simulink model "HIL_HallTesting"  (R2024b)
settings: Solver=ode23t  StartTime=0.0  StopTime=Inf  FixedStep=1e-2  RelTol=1e-3
undefined symbols (not defined in the file): DiscIntNeverNeededParam
libraries: fl_lib x6, nesl_utility x4, instrumentseriallib x3, svdutilitieslib x2
settings Model: SimulationMode=accelerator  Creator=luigi  LastModifiedBy=luigi
settings HardwareCC: ProdBitPerLong=64  ProdHWDeviceType=Intel->x86-64 (Linux 64)
settings SFSimCC: SimCustomCompilerFlags="CFLAGS  = -g -Wall -std=c99 -D_POSIX_SOURCE -D_GNU_SOURCE LDFLAGS = -lpthread -lrt"
settings RTWCC: Description=Simulink Desktop Real-Time  SystemTargetFile=sldrt.tlc  GenerateMakefile=off  TemplateMakefile=sldrt.tmf  CustomInclude=/usr/include/linux/  RTWCompilerOptimization=on
settings RTWCC: CustomHeaderCode=|
  | #include "time.h"
  | #include "stdint.h"
settings CodeAppCC: MaxIdLength=95
settings SimulinkDesktopRealTimeCC: TargetLibSuffix=_sldrt.a  TargetPreCompLibLocation=/usr/local/MATLAB/R2024b/toolbox/sldrt/lib/glnxa64  CodeReplacementLibrary=GNU C99 extensions  ParMdlRefBuildCompliant=on

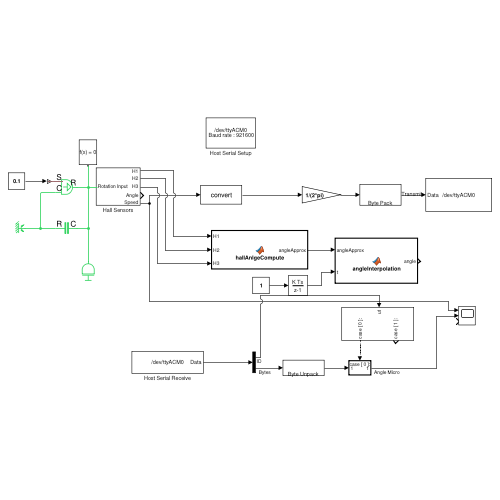
[thumbnail: Simulink's stored preview of the top-level diagram]
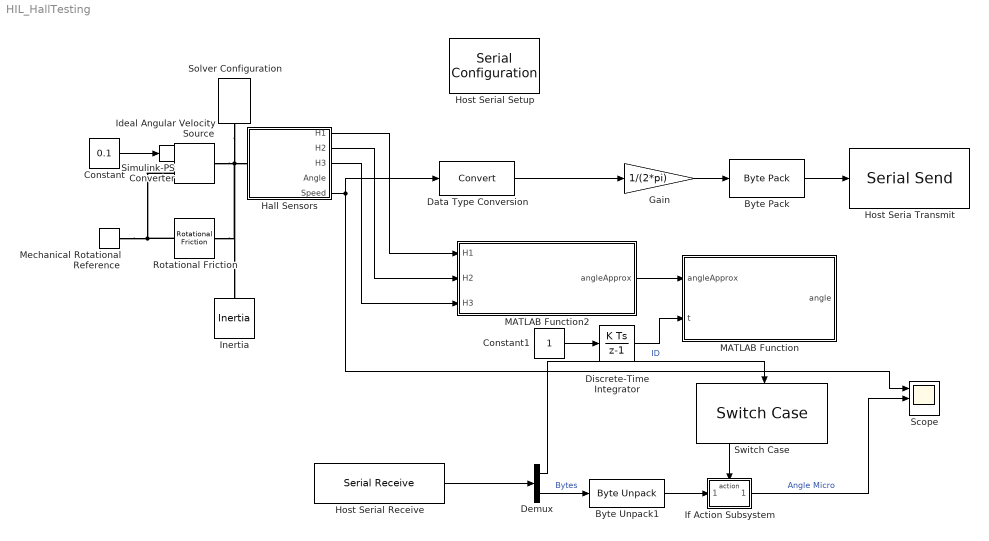
== system HIL_HallTesting ==
  Byte Pack : svdutilitieslib/Byte Pack  maskPackedDataType=uint8  datatypes={'single'}  byteAlign=1  blockPlatform=arduinoert
      settings: LibrarySourceBlock=mcblib/Signal Management/Byte Pack
  Byte Unpack1 : svdutilitieslib/Byte Unpack  dimensions={[1]}  datatypes={'single'}  byteAlign=1  blockPlatform=arduinoert
      settings: LibrarySourceBlock=mcblib/Signal Management/Byte Unpack
  Constant : Constant  Value=0.1
  Constant1 : Constant
  Data Type Conversion : DataTypeConversion  SaturateOnIntegerOverflow=off  RndMeth=Floor
  Demux : Demux  Outputs=[1 4]
  Discrete-Time Integrator : DiscreteIntegrator  SampleTime=-1  ICPrevOutput=DiscIntNeverNeededParam  ICPrevScaledInput=DiscIntNeverNeededParam
  Gain : Gain  Gain=1/(2*pi)
  Hall Sensors : Subsystem
  Host Seria Transmit : instrumentseriallib/Serial Send  PortSel=/dev/ttyACM0  Port=/dev/ttyACM0  ComPort=/dev/ttyACM0  Header=6  Terminator=<none>  CustomTerminator='EOF'  EnableBlockingMode=off  SimulateUsing=Interpreted execution  BlockInModel=on  aMode=5
      settings: LibrarySourceBlock=mcblib/Protection and Diagnostics/Host Serial Transmit
  Host Serial Receive : instrumentseriallib/Serial Receive  PortSel=/dev/ttyACM0  Port=/dev/ttyACM0  ComPort=/dev/ttyACM0  DataType=uint8  SaveDataType=uint8  ToggleHeader=off  Header='S'  ToggleDataSize=on  DataSize=5  ToggleTerminator=on  Terminator=Custom terminator  CustomTerminator='EOF'  InputFormat=Column major  EnableBlockingMode=on  ActionDataUnavailable=Output last received value  ActionWhenDataUnavailable=Output last received value  CustomValue=0  SampleTime=1e-2  SimulateUsing=Interpreted execution  BlockInModel=on  aMode=5
      settings: LibrarySourceBlock=mcblib/Protection and Diagnostics/Host Serial Receive
  Host Serial Setup : instrumentseriallib/Serial Configuration  Priority=-99  PortSel=/dev/ttyACM0  Port=/dev/ttyACM0  ComPort=/dev/ttyACM0  BaudRate=921600  DataBits=8  Parity=none  StopBits=1  ByteOrder=little-endian  FlowControl=none  Timeout=10  SimulateUsing=Interpreted execution  BlockInModel=on  aMode=5
      settings: LibrarySourceBlock=mcblib/Protection and Diagnostics/Host Serial Setup
  Ideal Angular Velocity Source : fl_lib/Mechanical/Mechanical Sources/Ideal Angular Velocity Source
  If Action Subsystem : Subsystem  TreatAsAtomicUnit=on
  Inertia : fl_lib/Mechanical/Rotational Elements/Inertia  inertia=0.1 kg*m^2  num_ports=foundation.enum.numPorts2.one  w_specify=off  w_priority=High  w=0 rad/s  w_nominal_specify=off  w_nominal_value=1  w_nominal_unit=rad/s  t_specify=off  t_priority=None  t=0 N*m  t_nominal_specify=off  t_nominal_value=1  t_nominal_unit=N*m
  MATLAB Function : MATLAB Function  TreatAsAtomicUnit=on  SystemSampleTime=1e-3
  MATLAB Function2 : MATLAB Function  TreatAsAtomicUnit=on
  Mechanical Rotational Reference : fl_lib/Mechanical/Rotational Elements/Mechanical Rotational Reference
  Rotational Friction : fl_lib/Mechanical/Rotational Elements/Rotational Friction  brkwy_trq=0.05 N*m  brkwy_vel=0.1 rad/s  Col_trq=0.01 N*m  visc_coef=0.01 N*m*s/rad  w_specify=off  w_priority=None  w=0 rad/s  w_nominal_specify=off  w_nominal_value=1  w_nominal_unit=rad/s  t_specify=off  t_priority=None  t=0 N*m  t_nominal_specify=off  t_nominal_value=1  t_nominal_unit=N*m
  Scope : Scope  NumInputPorts=3
  Simulink-PS Converter : nesl_utility/Simulink-PS Converter  PhysicalDomain=network_engine_domain  SubClassName=ps_input  LeftPortType=input  RightPortType=output  PseudoPeriodic=off  Frequencies=[]  NoiseDistribution=none  NoiseParameters=[]  Unit=1  AffineConversion=off  FilteringAndDerivatives=provide  SimscapeFilterOrder=1  InputFilterTimeConstant=0.001  UdotUserProvided=0
  Solver Configuration : nesl_utility/Solver Configuration  PhysicalDomain=network_engine_domain  SubClassName=solver  LeftPortType=input  RightPortType=generic  Tones=[]  Harmonics=[]  SimulateNoise=off  Profile=off  UseLocalSampling=off  EnableSwitchedLinearOptims=on  FrequencyDomain=off  UseCCode=off  RelTol=0.001  AbsTol=0.001  MinStep=1e-09  ToWorkspace=off  RevertToSquareIcSolve=off  NumHomotopyIterations=100  PhasorMode=off  PhasorModeNumHarmonics=1  ConsistencySolver=NEWTON_XTOL_AFTER_FTOL  IndexReductionMethod=DerivativeReplacement  DoDC=off  ResidualTolerance=1e-09  ConsistencyTolSource=GLOBAL  ConsistencyAbsTol=0.001  ConsistencyRelTol=0.001  ConsistencyTolFactor=0.001  UseLocalSolver=off  LocalSolverChoice=NE_BACKWARD_EULER_ADVANCER  ResolveIndetEquations=on  FunctionEvalNumThread=1  LocalSolverSampleTime=0.001  DoFixedCost=off  MaxNonlinIter=3  MaxModeIter=2  ComputeImpulses=off  ImpulseIterations=2  LinearAlgebra=auto  LinearAlgebraNumThread=0  EquationFormulation=NE_TIME_EF  DelaysMemoryBudget=1024  AutomaticFiltering=on  FilteringTimeConstant=0.001  PartitionStorageMethod=AS_NEEDED  PartitionMemoryBudget=1024  PartitionMethod=ROBUST  MultibodyUseLocalSolver=off  MultibodyLocalSolverChoice=ODE1  MultibodyLocalSolverSampleTime=0.001
  Switch Case : SwitchCase  CaseConditions={0,1}  ShowDefaultCase=off
  wires:
  Constant/1 -> Simulink-PS Converter/1
  Hall Sensors/1(H1) -> MATLAB Function2/1(H1)
  Hall Sensors/2(H2) -> MATLAB Function2/2(H2)
  Hall Sensors/3(H3) -> MATLAB Function2/3(H3)
  Discrete-Time Integrator/1 -> MATLAB Function/2(t)
  MATLAB Function2/1(angleApprox) -> MATLAB Function/1(angleApprox)
  Host Serial Receive/1 -> Demux/1
  Demux/1 -> Switch Case/1  "ID"
  Switch Case/1 -> If Action Subsystem/Action
  Byte Unpack1/1 -> If Action Subsystem/1(In1)
  Demux/2 -> Byte Unpack1/1  "Bytes"
  If Action Subsystem/1(Out1) -> Scope/2  "Angle Micro"
  Constant1/1 -> Discrete-Time Integrator/1
  Hall Sensors/5(Speed) -> Data Type Conversion/1, Scope/1
  Byte Pack/1 -> Host Seria Transmit/1
  Gain/1 -> Byte Pack/1
  Data Type Conversion/1 -> Gain/1
  connections:
  Mechanical Rotational Reference/LConn1 -- Ideal Angular Velocity Source/RConn2 -- Rotational Friction/LConn1
  Ideal Angular Velocity Source/RConn1 -- Simulink-PS Converter/RConn1
  Solver Configuration/RConn1 -- Ideal Angular Velocity Source/LConn1 -- Rotational Friction/RConn1 -- Inertia/LConn1 -- Hall Sensors/LConn1

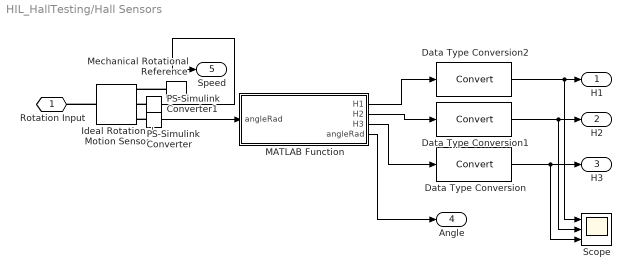
== system HIL_HallTesting/Hall Sensors ==
  Data Type Conversion : DataTypeConversion  SaturateOnIntegerOverflow=off  RndMeth=Floor
  Data Type Conversion1 : DataTypeConversion  SaturateOnIntegerOverflow=off  RndMeth=Floor
  Data Type Conversion2 : DataTypeConversion  SaturateOnIntegerOverflow=off  RndMeth=Floor
  Ideal Rotational Motion Sensor : fl_lib/Mechanical/Mechanical Sensors/Ideal Rotational Motion Sensor  reference=foundation.enum.MeasurementReference.difference  acceleration_port=false  velocity_port=true  position_port=true  wrap_angle=true  offset=0 rad
  MATLAB Function : MATLAB Function  TreatAsAtomicUnit=on
  Mechanical Rotational Reference : fl_lib/Mechanical/Rotational Elements/Mechanical Rotational Reference
  PS-Simulink Converter : nesl_utility/PS-Simulink Converter  PhysicalDomain=network_engine_domain  SubClassName=ps_output  LeftPortType=input  RightPortType=output  PseudoPeriodic=off  Frequencies=[]  VectorFormat=inherit  Unit=inherit  AffineConversion=off
  PS-Simulink Converter1 : nesl_utility/PS-Simulink Converter  PhysicalDomain=network_engine_domain  SubClassName=ps_output  LeftPortType=input  RightPortType=output  PseudoPeriodic=off  Frequencies=[]  VectorFormat=inherit  Unit=inherit  AffineConversion=off
  Scope : Scope  NumInputPorts=3
  Rotation Input : PMIOPort  Side=Left
  H1 : Outport  OutDataTypeStr=uint8
  H2 : Outport  Port=2  OutDataTypeStr=uint8
  H3 : Outport  Port=3  OutDataTypeStr=uint8
  Angle : Outport  Port=4  OutDataTypeStr=double
  Speed : Outport  Port=5  OutDataTypeStr=double
  wires:
  MATLAB Function/2(H2) -> Data Type Conversion1/1
  MATLAB Function/3(H3) -> Data Type Conversion/1
  PS-Simulink Converter/1 -> MATLAB Function/1("angleRad ")
  MATLAB Function/1(H1) -> Data Type Conversion2/1
  Data Type Conversion/1 -> Scope/3, H3/1
  Data Type Conversion1/1 -> Scope/2, H2/1
  Data Type Conversion2/1 -> H1/1, Scope/1
  MATLAB Function/4(angleRad) -> Angle/1
  PS-Simulink Converter1/1 -> Speed/1
  connections:
  PS-Simulink Converter/LConn1 -- Ideal Rotational Motion Sensor/RConn3
  Ideal Rotational Motion Sensor/LConn1 -- Rotation Input/RConn1
  Mechanical Rotational Reference/LConn1 -- Ideal Rotational Motion Sensor/RConn1
  PS-Simulink Converter1/LConn1 -- Ideal Rotational Motion Sensor/RConn2

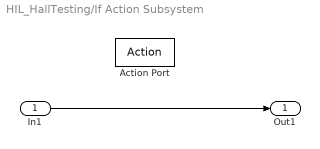
== system HIL_HallTesting/If Action Subsystem ==
  In1 : Inport
  Action Port : ActionPort  ActionPortLabel=case [ 0 ]:
  Out1 : Outport
  wires:
  In1/1 -> Out1/1

== matlab function HIL_HallTesting/Hall Sensors/MATLAB Function ==
  settings: updateMethod=DISCRETE  sampleTime=1e-3
  data: angleRad input; H1 output; H2 output; H3 output; angleRad output
function [H1, H2, H3, angleRad] = angle2hall(angleRad)

HALL_DEGREES = pi/3;

% The LUT was built according to maxon catalogue page 67
% https://online.flippingbook.com/view/398826/67/#zoom=true

HALL_OUT_LUT_60 = [1,0,1;1,0,0;1,1,0;0,1,0;0,1,1;0,0,1];

%angleDeg = angleRad * (180/pi);
% angleRad = 2*pi - angleRad  ;

angleRad = angleRad * 8;
angleRad = mod(angleRad, 2*pi);

anglePosition = round(angleRad/HALL_DEGREES) + 1;

if anglePosition > 6
    anglePosition = 1;
end

if anglePosition < 1
    anglePosition = 1;
end

H3 = HALL_OUT_LUT_60(anglePosition,1);
H2 = HALL_OUT_LUT_60(anglePosition,2);
H1 = HALL_OUT_LUT_60(anglePosition,3);




end

== matlab function HIL_HallTesting/MATLAB Function2 ==
  settings: updateMethod=DISCRETE  sampleTime=1e-3
  data: H1 input uint8; H2 input uint8; H3 input uint8; angleApprox output
function angleApprox  = hallAnlgeCompute( H1, H2, H3)

    % HALL_OUT_LUT_60 = [1,0,1;1,0,0;1,1,0;0,1,0;0,1,1;0,0,1];
    
    hallReading = bitor(bitshift(H2, 1), bitshift(H3, 2));
    hallReading = bitor(hallReading, bitshift(H1, 0));

    angleApprox = 0;
    switch hallReading
        case 0b101
            angleApprox = 0;
        case 0b100
            angleApprox = 0;
        case 0b110
            angleApprox = 2*pi/3;
        case 0b010
            angleApprox = 2*pi/3;
        case 0b011
            angleApprox = 4*pi/3;
        case 0b001
            angleApprox = 4*pi/3;
    end

end

== matlab function HIL_HallTesting/MATLAB Function ==
  data: angleApprox input; angle output; t input
function angle = angleInterpolation(angleApprox, t)

persistent oldAngle
persistent oldTime
persistent oldSpeed

if isempty(oldAngle)
    oldAngle = 0;
end
if isempty(oldTime)
    oldTime = 0;
end
if isempty(oldSpeed)
    oldSpeed = 0;
end

if oldAngle ~= angleApprox 
    oldSpeed = (2*pi/3) / abs(t - oldTime);
    oldTime = t;
    oldAngle = angleApprox;
end

angle = oldAngle + oldSpeed * (t - oldTime);
